simulink model "SSR_naponski"  (R2023b)
settings: Solver=VariableStepAuto  StartTime=0.0  StopTime=10  RelTol=1e-3
undefined symbols (not defined in the file or in its folder): A_ccm, A_dcm, B_ccm, B_dcm, C_ccm, C_dcm, CCM_tf_d_den, CCM_tf_d_num, CCM_tf_i1_den, CCM_tf_i1_num, D0_ccm, D0_dcm, D_ccm, D_dcm, DCM_tf_d_den, DCM_tf_d_num, DCM_tf_i1_den, DCM_tf_i1_num, I10_ccm, I10_dcm, IL0_ccm, IL0_dcm, L, T, Ubat0_ccm, Ubat0_dcm, Upv0
libraries: simulink_extras x10, dspstat3 x4
settings Model: Creator=teo  LastModifiedBy=teo

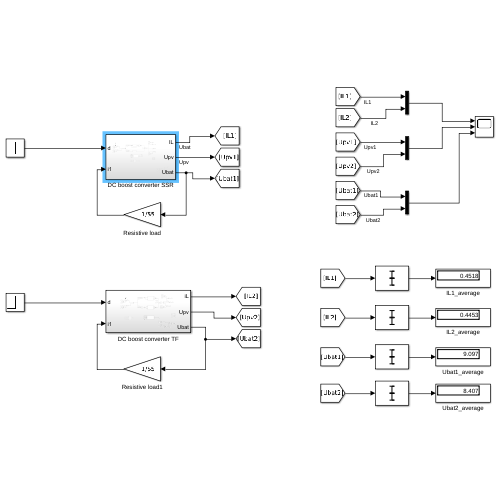
[thumbnail: Simulink's stored preview of the top-level diagram]
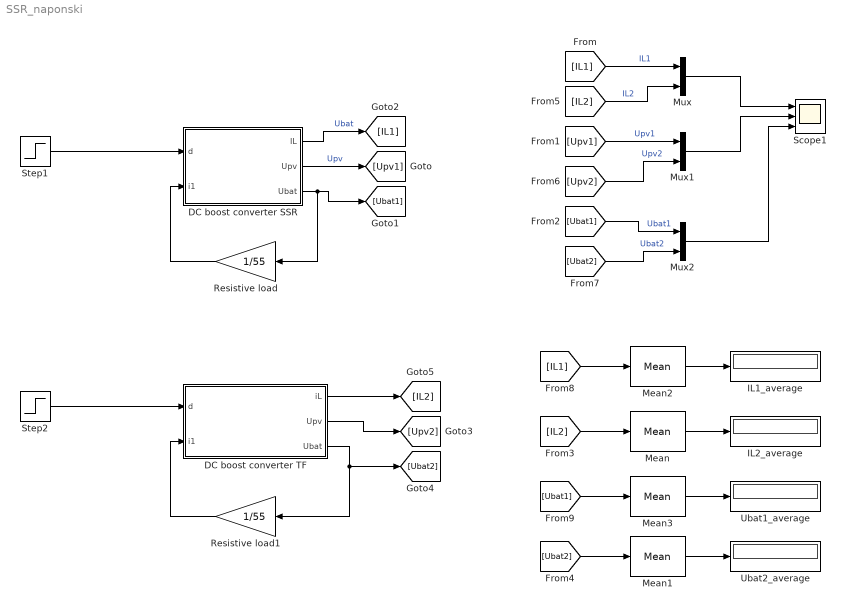
== system SSR_naponski ==
  DC boost converter SSR : Subsystem
  DC boost converter TF : Subsystem
  IL1_average : Display
  IL2_average : Display
  Mean{,1..3} (4 alike) : dspstat3/Mean  run=off  InputProcessing=Columns as channels (frame based)  reset_popup=None  directionMode=Entire input  dimension=1  roiEnable=off  roiType=Rectangles  roiPortion=Entire ROI  roiOutput=Individual statistics for each ROI  roiFlag=off  roundingMode=Floor  overflowMode=off  outputDataTypeStr=Inherit: Same as accumulator  outputMin=[]  outputMax=[]  outputLastDataTypeStr=Inherit: Same as accumulator
  Mux : Mux  Inputs=2
  Mux1 : Mux  Inputs=2
  Mux2 : Mux  Inputs=2
  Resistive load : Gain  Gain=1/55
  Resistive load1 : Gain  Gain=1/55
  Scope1 : Scope  NumInputPorts=3
  Step1 : Step  Time=5  Before=0.4  After=0.75  SampleTime=0
  Step2 : Step  Time=5  Before=0.4  After=0.75  SampleTime=0
  Ubat1_average : Display
  Ubat2_average : Display
  wires:
  Resistive load/1 -> DC boost converter SSR/2(i1)
  DC boost converter SSR/2(Upv) -> [Upv1]  "Upv"
  DC boost converter SSR/3(Ubat) -> Resistive load/1, [Ubat1]
  DC boost converter SSR/1(IL) -> [IL1]  "Ubat"
  Mean/1 -> IL2_average/1
  [IL2] -> Mean/1
  [Ubat2] -> Mean1/1
  Mean1/1 -> Ubat2_average/1
  Step2/1 -> DC boost converter TF/1(d)
  DC boost converter TF/3(Ubat) -> [Ubat2], Resistive load1/1
  Resistive load1/1 -> DC boost converter TF/2(i1)
  DC boost converter TF/1(iL) -> [IL2]
  DC boost converter TF/2(Upv) -> [Upv2]
  [IL1] -> Mux/1  "IL1"
  [IL2] -> Mux/2  "IL2"
  [Upv1] -> Mux1/1  "Upv1"
  [Upv2] -> Mux1/2  "Upv2"
  Mux/1 -> Scope1/1
  Mux1/1 -> Scope1/2
  [Ubat1] -> Mux2/1  "Ubat1"
  Mux2/1 -> Scope1/3
  [Ubat2] -> Mux2/2  "Ubat2"
  Mean2/1 -> IL1_average/1
  [IL1] -> Mean2/1
  [Ubat1] -> Mean3/1
  Mean3/1 -> Ubat1_average/1
  Step1/1 -> DC boost converter SSR/1(d)

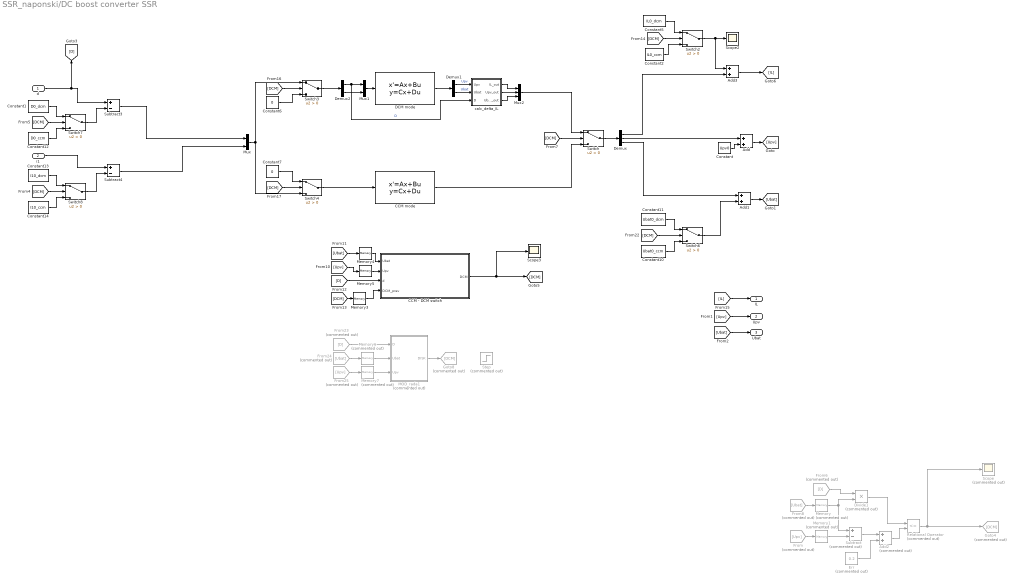
== system SSR_naponski/DC boost converter SSR ==
  d : Inport
  i1 : Inport  Port=2
  Add : Sum
  Add1 : Sum
  Add2 : Sum  Commented=on
  Add3 : Sum
  CCM - DCM switch : Subsystem
  CCM mode : StateSpace  A=A_ccm  B=B_ccm  C=C_ccm  D=D_ccm  InitialCondition=0  ContinuousStateAttributes="\"\""
  Constant : Constant  Value=Upv0
  Constant1 : Constant  Value=D0_dcm
  Constant10 : Constant  Value=Ubat0_ccm
  Constant11 : Constant  Value=Ubat0_dcm
  Constant12 : Constant  Value=D0_ccm
  Constant13 : Constant  Value=I10_dcm
  Constant14 : Constant  Value=I10_ccm
  Constant2 : Constant  Value=IL0_ccm
  Constant5 : Constant  Value=IL0_dcm
  Constant6 : Constant  Value=0
  Constant7 : Constant  Value=0
  DCM mode : StateSpace  A=A_dcm  B=B_dcm  C=C_dcm  D=D_dcm  InitialCondition=0  ContinuousStateAttributes="\"\""
  Demux : Demux  Outputs=3
  Demux1 : Demux  Outputs=2
  Demux2 : Demux  Outputs=2
  Divide1 : Product  Commented=on  Inputs=**
  Err : Constant  Commented=on  Value=0.2
  From : From  Commented=on  GotoTag=Upv
  From23 : From  Commented=on  GotoTag=D
  From24 : From  Commented=on  GotoTag=Ubat
  From25 : From  Commented=on  GotoTag=Upv
  From6 : From  Commented=on  GotoTag=D
  From8 : From  Commented=on  GotoTag=Ubat
  Goto4 : Goto  Commented=on  GotoTag=DCM
  Goto8 : Goto  Commented=on  GotoTag=DCM
  MOD_rada1 : Subsystem  Commented=on
  Memory{,1,6..7} (4 alike) : Memory  Commented=on
  Memory3 : Memory
  Memory4 : Memory
  Memory5 : Memory
  Mux : Mux  Inputs=2
  Mux1 : Mux  Inputs=2
  Mux2 : Mux  Inputs=3
  Relational Operator : RelationalOperator  Commented=on  Operator=<=  OutDataTypeStr=boolean  RndMeth=Simplest  InputSameDT=off
  Scope : Scope  Commented=on
  Scope2 : Scope
  Scope3 : Scope
  Step : Step  Commented=on  Time=5  SampleTime=0
  Subtract : Sum  Commented=on  Inputs=+-
  Subtract3 : Sum  Inputs=+-
  Subtract4 : Sum  Inputs=+-
  Switch{,2..4,6..8} (7 alike) : Switch  Criteria=u2 > Threshold  SaturateOnIntegerOverflow=off  InputSameDT=off
  calc_delta_IL : Subsystem
  IL : Outport
  Upv : Outport  Port=2
  Ubat : Outport  Port=3
  wires:
  From6/1 -> Divide1/1
  Add/1 -> [Upv]
  Add1/1 -> [Ubat]
  [DCM] -> Switch/2
  Relational Operator/1 -> Goto4/1, Scope/1
  Switch/1 -> Demux/1
  Demux1/1 -> calc_delta_IL/1(Upv)  "Upv"
  Demux1/2 -> calc_delta_IL/2(Ubat)  "Ubat"
  Demux2/1 -> calc_delta_IL/3(D), Mux1/1  "D"
  Demux2/2 -> Mux1/2
  calc_delta_IL/1(IL_out) -> Mux2/1
  calc_delta_IL/2(Upv_out) -> Mux2/2
  calc_delta_IL/3(Ubat_out) -> Mux2/3
  Demux/3 -> Add1/1
  Constant/1 -> Add/2
  Demux/2 -> Add/1
  Constant5/1 -> Switch2/1
  Constant2/1 -> Switch2/3
  [DCM] -> Switch2/2
  Add3/1 -> [IL]
  Mux1/1 -> DCM mode/1
  DCM mode/1 -> Demux1/1
  CCM mode/1 -> Switch/3
  Mux2/1 -> Switch/1
  [Ubat] -> Ubat/1
  [Upv] -> Upv/1
  [IL] -> IL/1
  Switch3/1 -> Demux2/1
  Switch4/1 -> CCM mode/1
  [DCM] -> Switch3/2
  [DCM] -> Switch4/2
  Constant6/1 -> Switch3/3
  Constant7/1 -> Switch4/1
  Mux/1 -> Switch4/3, Switch3/1
  Constant11/1 -> Switch6/1
  Constant10/1 -> Switch6/3
  [DCM] -> Switch6/2
  Switch6/1 -> Add1/2
  Memory5/1 -> CCM - DCM switch/2(Upv)
  Memory3/1 -> CCM - DCM switch/4(DCM_prev)
  [DCM] -> Memory3/1
  [Ubat] -> Memory4/1
  [D] -> CCM - DCM switch/3(d)
  Memory4/1 -> CCM - DCM switch/1(Ubat)
  CCM - DCM switch/1(DCM) -> Scope3/1, [DCM]
  [Upv] -> Memory5/1
  From23/1 -> MOD_rada1/1(D)
  MOD_rada1/1(DISK) -> Goto8/1
  Memory6/1 -> MOD_rada1/2(Ubat)
  From25/1 -> Memory7/1
  Memory7/1 -> MOD_rada1/3(Upv)
  From24/1 -> Memory6/1
  Switch2/1 -> Add3/1, Scope2/1
  Demux/1 -> Add3/2
  [DCM] -> Switch7/2
  Constant14/1 -> Switch8/3
  Switch7/1 -> Subtract3/2
  Constant13/1 -> Switch8/1
  Constant12/1 -> Switch7/3
  Constant1/1 -> Switch7/1
  [DCM] -> Switch8/2
  Switch8/1 -> Subtract4/2
  Subtract3/1 -> Mux/1
  Subtract4/1 -> Mux/2
  i1/1 -> Subtract4/1
  d/1 -> [D], Subtract3/1
  From8/1 -> Memory/1
  From/1 -> Memory1/1
  Memory1/1 -> Subtract/2
  Memory/1 -> Subtract/1, Divide1/2
  Err/1 -> Add2/2
  Subtract/1 -> Add2/1
  Divide1/1 -> Relational Operator/1
  Add2/1 -> Relational Operator/2

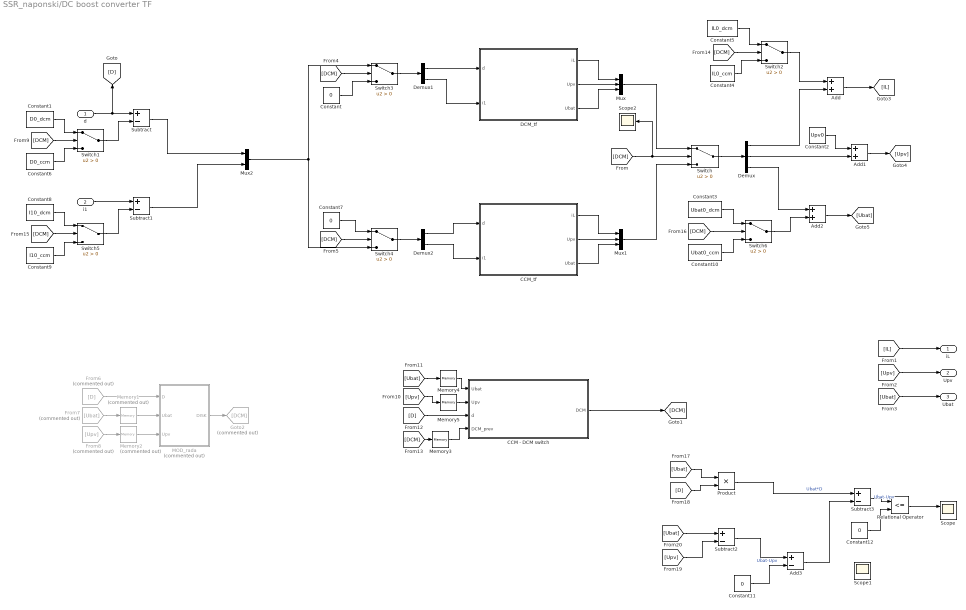
== system SSR_naponski/DC boost converter TF ==
  d : Inport
  i1 : Inport  Port=2
  Add : Sum
  Add1 : Sum
  Add2 : Sum
  Add3 : Sum  Inputs=+-
  CCM - DCM switch : Subsystem
  CCM_tf : Subsystem
  Constant{,7,11..12} (4 alike) : Constant  Value=0
  Constant1 : Constant  Value=D0_dcm
  Constant10 : Constant  Value=Ubat0_ccm
  Constant2 : Constant  Value=Upv0
  Constant3 : Constant  Value=Ubat0_dcm
  Constant4 : Constant  Value=IL0_ccm
  Constant5 : Constant  Value=IL0_dcm
  Constant6 : Constant  Value=D0_ccm
  Constant8 : Constant  Value=I10_dcm
  Constant9 : Constant  Value=I10_ccm
  DCM_tf : Subsystem
  Demux : Demux  Outputs=3
  Demux1 : Demux  Outputs=2
  Demux2 : Demux  Outputs=2
  From6 : From  Commented=on  GotoTag=D
  From7 : From  Commented=on  GotoTag=Ubat
  From8 : From  Commented=on  GotoTag=Upv
  Goto2 : Goto  Commented=on  GotoTag=DCM
  MOD_rada : Subsystem  Commented=on
  Memory1 : Memory  Commented=on
  Memory2 : Memory  Commented=on
  Memory3 : Memory
  Memory4 : Memory
  Memory5 : Memory
  Mux : Mux  Inputs=3
  Mux1 : Mux  Inputs=3
  Mux2 : Mux  Inputs=2
  Product : Product
  Relational Operator : RelationalOperator  Operator=<=  OutDataTypeStr=boolean  RndMeth=Simplest  InputSameDT=off
  Scope : Scope  NumInputPorts=2
  Scope1 : Scope
  Scope2 : Scope
  Subtract{,1..3} (4 alike) : Sum  Inputs=+-
  Switch{,1..6} (7 alike) : Switch  Criteria=u2 > Threshold  SaturateOnIntegerOverflow=off  InputSameDT=off
  iL : Outport
  Upv : Outport  Port=2
  Ubat : Outport  Port=3
  wires:
  Add1/1 -> [Upv]
  Add2/1 -> [Ubat]
  Add/1 -> [IL]
  [D] -> CCM - DCM switch/3(d)
  DCM_tf/2(Upv) -> Mux/2
  DCM_tf/1(iL) -> Mux/1
  DCM_tf/3(Ubat) -> Mux/3
  CCM_tf/1(iL) -> Mux1/1
  CCM_tf/2(Upv) -> Mux1/2
  CCM_tf/3(Ubat) -> Mux1/3
  Mux1/1 -> Switch/3
  Mux/1 -> Switch/1
  [DCM] -> Switch/2, Scope2/1
  Switch/1 -> Demux/1
  Constant5/1 -> Switch2/1
  Constant4/1 -> Switch2/3
  [DCM] -> Switch2/2
  Switch2/1 -> Add/1
  Demux/1 -> Add/2
  Demux/2 -> Add1/2
  Constant2/1 -> Add1/1
  Demux/3 -> Add2/1
  [IL] -> iL/1
  [Upv] -> Upv/1
  [Ubat] -> Ubat/1
  Constant6/1 -> Switch1/3
  Constant1/1 -> Switch1/1
  [DCM] -> Switch1/2
  Switch3/1 -> Demux1/1
  Demux1/1 -> DCM_tf/1(d)
  Demux1/2 -> DCM_tf/2(i1)
  Demux2/1 -> CCM_tf/1(d)
  Demux2/2 -> CCM_tf/2(i1)
  Switch4/1 -> Demux2/1
  Mux2/1 -> Switch4/3, Switch3/1
  Constant/1 -> Switch3/3
  Constant7/1 -> Switch4/1
  [DCM] -> Switch3/2
  [DCM] -> Switch4/2
  CCM - DCM switch/1(DCM) -> [DCM]
  MOD_rada/1(DISK) -> Goto2/1
  From6/1 -> MOD_rada/1(D)
  Memory1/1 -> MOD_rada/2(Ubat)
  From7/1 -> Memory1/1
  Memory2/1 -> MOD_rada/3(Upv)
  From8/1 -> Memory2/1
  [Ubat] -> Memory4/1
  [Upv] -> Memory5/1
  Memory5/1 -> CCM - DCM switch/2(Upv)
  Memory4/1 -> CCM - DCM switch/1(Ubat)
  d/1 -> [D], Subtract/1
  Switch1/1 -> Subtract/2
  [DCM] -> Switch5/2
  Constant8/1 -> Switch5/1
  Constant9/1 -> Switch5/3
  Switch5/1 -> Subtract1/2
  Subtract1/1 -> Mux2/2
  i1/1 -> Subtract1/1
  [DCM] -> Memory3/1
  Memory3/1 -> CCM - DCM switch/4(DCM_prev)
  Switch6/1 -> Add2/2
  Constant3/1 -> Switch6/1
  Constant10/1 -> Switch6/3
  [DCM] -> Switch6/2
  Subtract/1 -> Mux2/1
  [Ubat] -> Product/1
  [D] -> Product/2
  [Ubat] -> Subtract2/1
  [Upv] -> Subtract2/2
  Subtract2/1 -> Add3/1  "Ubat-Upv"
  Product/1 -> Subtract3/1  "Ubat*D"
  Constant11/1 -> Add3/2
  Add3/1 -> Subtract3/2
  Subtract3/1 -> Relational Operator/1  "Ubat-Upv"
  Constant12/1 -> Relational Operator/2
  Relational Operator/1 -> Scope/1

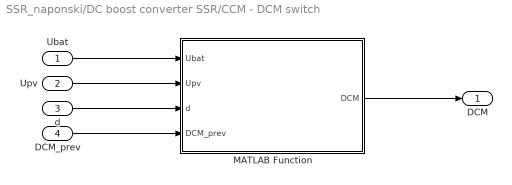
== system SSR_naponski/DC boost converter SSR/CCM - DCM switch ==
  Ubat : Inport
  Upv : Inport  Port=2
  d : Inport  Port=3
  DCM_prev : Inport  Port=4
  MATLAB Function : MATLAB Function  TreatAsAtomicUnit=on
  DCM : Outport
  wires:
  MATLAB Function/1(DCM) -> DCM/1
  Ubat/1 -> MATLAB Function/1(Ubat)
  Upv/1 -> MATLAB Function/2(Upv)
  d/1 -> MATLAB Function/3(d)
  DCM_prev/1 -> MATLAB Function/4(DCM_prev)

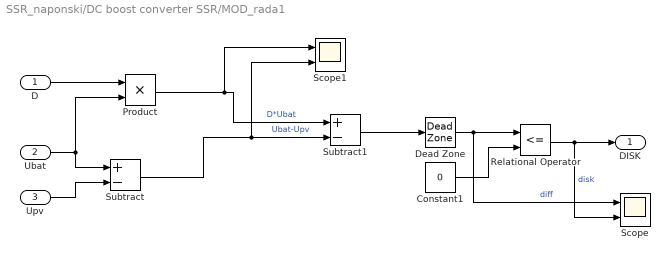
== system SSR_naponski/DC boost converter SSR/MOD_rada1 ==
  D : Inport
  Ubat : Inport  Port=2
  Upv : Inport  Port=3
  Constant1 : Constant  Value=0
  Dead Zone : DeadZone  UpperValue=0
  Product : Product
  Relational Operator : RelationalOperator  Operator=<=  OutDataTypeStr=boolean  RndMeth=Simplest  InputSameDT=off
  Scope : Scope  NumInputPorts=2
  Scope1 : Scope  NumInputPorts=2
  Subtract : Sum  Inputs=+-
  Subtract1 : Sum  Inputs=+-
  DISK : Outport
  wires:
  Ubat/1 -> Product/2, Subtract/1
  Upv/1 -> Subtract/2
  Product/1 -> Scope1/1, Subtract1/1  "D*Ubat"
  D/1 -> Product/1
  Subtract/1 -> Scope1/2, Subtract1/2  "Ubat-Upv"
  Subtract1/1 -> Dead Zone/1
  Dead Zone/1 -> Scope/1, Relational Operator/1  "diff"
  Relational Operator/1 -> Scope/2, DISK/1  "disk"
  Constant1/1 -> Relational Operator/2

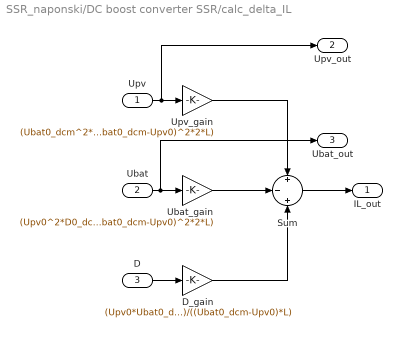
== system SSR_naponski/DC boost converter SSR/calc_delta_IL ==
  Upv : Inport
  Ubat : Inport  Port=2
  D : Inport  Port=3
  D_gain : Gain  Gain=(Upv0*Ubat0_dcm*D0_dcm*T)/((Ubat0_dcm-Upv0)*L)
  Sum : Sum  Inputs=+|-|+
  Ubat_gain : Gain  Gain=(Upv0^2*D0_dcm^2*T)/((Ubat0_dcm-Upv0)^2*2*L)
  Upv_gain : Gain  Gain=(Ubat0_dcm^2*D0_dcm^2*T)/((Ubat0_dcm-Upv0)^2*2*L)
  IL_out : Outport
  Upv_out : Outport  Port=2
  Ubat_out : Outport  Port=3
  wires:
  D/1 -> D_gain/1
  Upv/1 -> Upv_out/1, Upv_gain/1
  Ubat/1 -> Ubat_out/1, Ubat_gain/1
  Ubat_gain/1 -> Sum/2
  Upv_gain/1 -> Sum/1
  D_gain/1 -> Sum/3
  Sum/1 -> IL_out/1

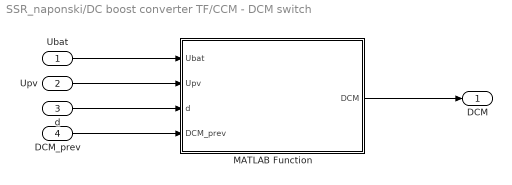
== system SSR_naponski/DC boost converter TF/CCM - DCM switch ==
  Ubat : Inport
  Upv : Inport  Port=2
  d : Inport  Port=3
  DCM_prev : Inport  Port=4
  MATLAB Function : MATLAB Function  TreatAsAtomicUnit=on
  DCM : Outport
  wires:
  MATLAB Function/1(DCM) -> DCM/1
  Ubat/1 -> MATLAB Function/1(Ubat)
  Upv/1 -> MATLAB Function/2(Upv)
  d/1 -> MATLAB Function/3(d)
  DCM_prev/1 -> MATLAB Function/4(DCM_prev)

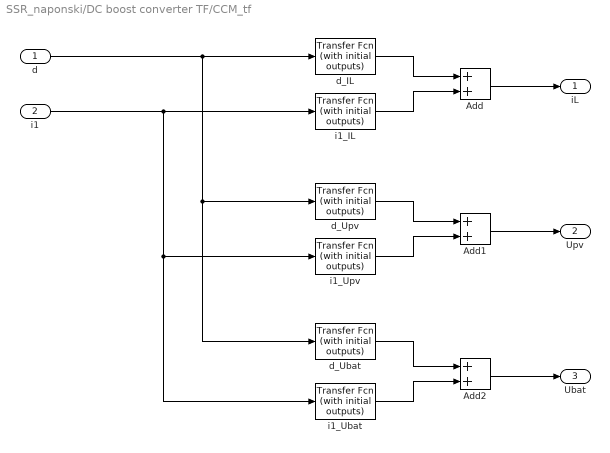
== system SSR_naponski/DC boost converter TF/CCM_tf ==
  d : Inport
  i1 : Inport  Port=2
  Add : Sum
  Add1 : Sum
  Add2 : Sum
  d_IL : simulink_extras/Additional Linear/Transfer Fcn (with initial outputs)  N=CCM_tf_d_num(1, :)  D=CCM_tf_d_den(:)  Y0=0  U0=0
  d_Ubat : simulink_extras/Additional Linear/Transfer Fcn (with initial outputs)  N=CCM_tf_d_num(3, :)  D=CCM_tf_d_den(:)  Y0=0  U0=0
  d_Upv : simulink_extras/Additional Linear/Transfer Fcn (with initial outputs)  N=CCM_tf_d_num(2, :)  D=CCM_tf_d_den(:)  Y0=0  U0=0
  i1_IL : simulink_extras/Additional Linear/Transfer Fcn (with initial outputs)  N=CCM_tf_i1_num(1, :)  D=CCM_tf_i1_den(:)  Y0=0  U0=0
  i1_Ubat : simulink_extras/Additional Linear/Transfer Fcn (with initial outputs)  N=CCM_tf_i1_num(3, :)  D=CCM_tf_i1_den(:)  Y0=0  U0=0
  i1_Upv : simulink_extras/Additional Linear/Transfer Fcn (with initial outputs)  N=CCM_tf_i1_num(2, :)  D=CCM_tf_i1_den(:)  Y0=0  U0=0
  iL : Outport
  Upv : Outport  Port=2
  Ubat : Outport  Port=3
  wires:
  d/1 -> d_Ubat/1, d_Upv/1, d_IL/1
  i1/1 -> i1_Ubat/1, i1_Upv/1, i1_IL/1
  d_IL/1 -> Add/1
  i1_IL/1 -> Add/2
  Add/1 -> iL/1
  d_Upv/1 -> Add1/1
  i1_Upv/1 -> Add1/2
  Add1/1 -> Upv/1
  d_Ubat/1 -> Add2/1
  i1_Ubat/1 -> Add2/2
  Add2/1 -> Ubat/1

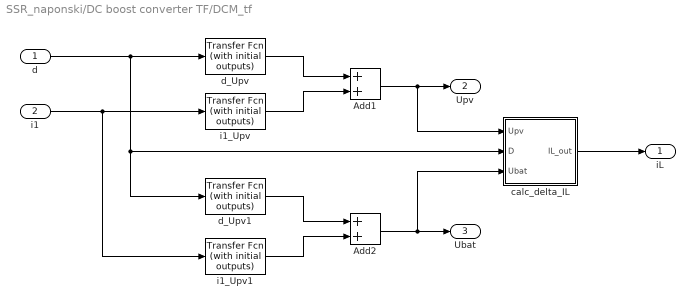
== system SSR_naponski/DC boost converter TF/DCM_tf ==
  d : Inport
  i1 : Inport  Port=2
  Add1 : Sum
  Add2 : Sum
  calc_delta_IL : Subsystem
  d_Upv : simulink_extras/Additional Linear/Transfer Fcn (with initial outputs)  N=DCM_tf_d_num(1, :)  D=DCM_tf_d_den(:)  Y0=0  U0=0
  d_Upv1 : simulink_extras/Additional Linear/Transfer Fcn (with initial outputs)  N=DCM_tf_d_num(2, :)  D=DCM_tf_d_den(:)  Y0=0  U0=0
  i1_Upv : simulink_extras/Additional Linear/Transfer Fcn (with initial outputs)  N=DCM_tf_i1_num(1, :)  D=DCM_tf_i1_den(:)  Y0=0  U0=0
  i1_Upv1 : simulink_extras/Additional Linear/Transfer Fcn (with initial outputs)  N=DCM_tf_i1_num(2, :)  D=DCM_tf_i1_den(:)  Y0=0  U0=0
  iL : Outport
  Upv : Outport  Port=2
  Ubat : Outport  Port=3
  wires:
  d_Upv/1 -> Add1/1
  i1_Upv/1 -> Add1/2
  Add1/1 -> calc_delta_IL/1(Upv), Upv/1
  d_Upv1/1 -> Add2/1
  i1_Upv1/1 -> Add2/2
  Add2/1 -> calc_delta_IL/3(Ubat), Ubat/1
  i1/1 -> i1_Upv1/1, i1_Upv/1
  d/1 -> d_Upv1/1, calc_delta_IL/2(D), d_Upv/1
  calc_delta_IL/1(IL_out) -> iL/1

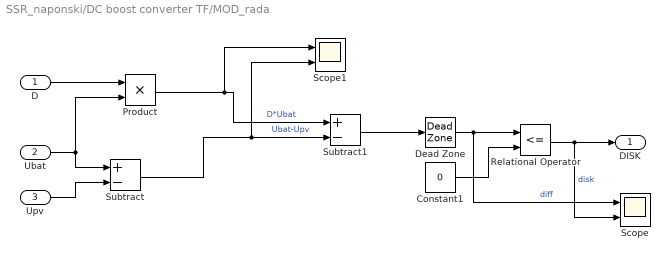
== system SSR_naponski/DC boost converter TF/MOD_rada ==
  D : Inport
  Ubat : Inport  Port=2
  Upv : Inport  Port=3
  Constant1 : Constant  Value=0
  Dead Zone : DeadZone  UpperValue=0
  Product : Product
  Relational Operator : RelationalOperator  Operator=<=  OutDataTypeStr=boolean  RndMeth=Simplest  InputSameDT=off
  Scope : Scope  NumInputPorts=2
  Scope1 : Scope  NumInputPorts=2
  Subtract : Sum  Inputs=+-
  Subtract1 : Sum  Inputs=+-
  DISK : Outport
  wires:
  Ubat/1 -> Product/2, Subtract/1
  Upv/1 -> Subtract/2
  Product/1 -> Scope1/1, Subtract1/1  "D*Ubat"
  D/1 -> Product/1
  Subtract/1 -> Scope1/2, Subtract1/2  "Ubat-Upv"
  Subtract1/1 -> Dead Zone/1
  Dead Zone/1 -> Scope/1, Relational Operator/1  "diff"
  Relational Operator/1 -> Scope/2, DISK/1  "disk"
  Constant1/1 -> Relational Operator/2

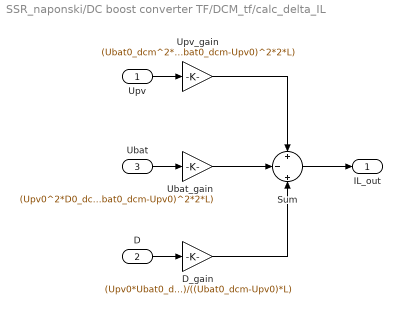
== system SSR_naponski/DC boost converter TF/DCM_tf/calc_delta_IL ==
  Upv : Inport
  D : Inport  Port=2
  Ubat : Inport  Port=3
  D_gain : Gain  Gain=(Upv0*Ubat0_dcm*D0_dcm*T)/((Ubat0_dcm-Upv0)*L)
  Sum : Sum  Inputs=+|-|+
  Ubat_gain : Gain  Gain=(Upv0^2*D0_dcm^2*T)/((Ubat0_dcm-Upv0)^2*2*L)
  Upv_gain : Gain  Gain=(Ubat0_dcm^2*D0_dcm^2*T)/((Ubat0_dcm-Upv0)^2*2*L)
  IL_out : Outport
  wires:
  D/1 -> D_gain/1
  Upv/1 -> Upv_gain/1
  Ubat/1 -> Ubat_gain/1
  Ubat_gain/1 -> Sum/2
  Upv_gain/1 -> Sum/1
  D_gain/1 -> Sum/3
  Sum/1 -> IL_out/1

== matlab function SSR_naponski/DC boost converter TF/CCM - DCM switch/MATLAB Function ==
  data: Ubat input; DCM output; Upv input; d input; DCM_prev input boolean
function DCM = fcn(Ubat, Upv, d, DCM_prev)
        
% Define sensitivity:
err = 1;

if DCM_prev % if in DCM
    if (d * Ubat >= Ubat - Upv + err)
        DCM = false;
    else
        DCM = DCM_prev;
    end
else % if in CCM
    if (d * Ubat <= Ubat - Upv - err)
        DCM = true;
    else
        DCM = DCM_prev;
    end
end

== matlab function SSR_naponski/DC boost converter SSR/CCM - DCM switch/MATLAB Function ==
  data: Ubat input; DCM output; Upv input; d input; DCM_prev input boolean
function DCM = fcn(Ubat, Upv, d, DCM_prev)
        
% Define sensitivity:
err = 1;

if DCM_prev % if in DCM
    if (d * Ubat >= Ubat - Upv + err)
        DCM = false;
    else
        DCM = DCM_prev;
    end
else % if in CCM
    if (d * Ubat <= Ubat - Upv - err)
        DCM = true;
    else
        DCM = DCM_prev;
    end
end
